simulink model "msim"  (R2024b)
settings: Solver=VariableStepAuto  StartTime=0.0  StopTime=10.0  RelTol=1e-3
values from neighbouring files (symbols this model uses):
  dtflin = c2d(tflin, Ts, "zoh")    [main.m]    (also in testdata.m)
  model_armax = armax(data_train, [na nb nc nk])    [main.m]
  model_arx = arx(data_train, [na nb nk])    [main.m]    (also in testdata.m)
settings Model: Creator=markminerov  LastModifiedBy=markminerov

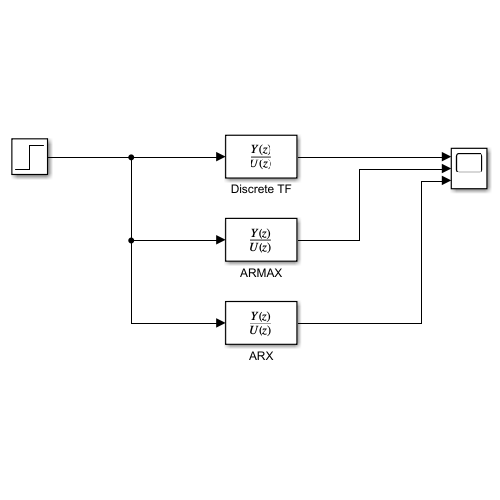
[thumbnail: Simulink's stored preview of the top-level diagram]
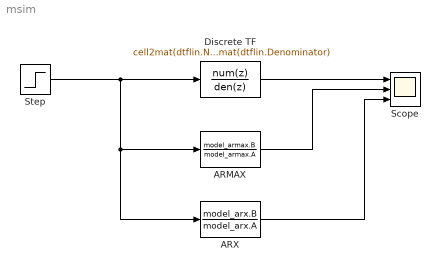
== system msim ==
  ARMAX : DiscreteTransferFcn  Numerator=model_armax.B  Denominator=model_armax.A
  ARX : DiscreteTransferFcn  Numerator=model_arx.B  Denominator=model_arx.A
  Discrete TF : DiscreteTransferFcn  Numerator=cell2mat(dtflin.Numerator)  Denominator=cell2mat(dtflin.Denominator)
  Scope : Scope  NumInputPorts=3
  Step : Step  SampleTime=0
  wires:
  Discrete TF/1 -> Scope/1
  Step/1 -> Discrete TF/1, ARX/1, ARMAX/1
  ARMAX/1 -> Scope/2
  ARX/1 -> Scope/3
